simulink model "test_polbereichsvorgabe"  (R2016b)
settings: Solver=FixedStepAuto  StartTime=0.0  StopTime=20.0  FixedStep=1e-3  RelTol=1e-3
values from neighbouring files (symbols this model uses):
  A_11 = matA_g_u(1:numMessg,1:numMessg)    [calcRedBEO.m]
  A_12 = matA_g_u(1:numMessg,numMessg+1:end)    [calcRedBEO.m]
  A_21 = matA_g_u(numMessg+1:end,1:numMessg)    [calcRedBEO.m]
  A_22 = matA_g_u(numMessg+1:end,numMessg+1:end)    [calcRedBEO.m]
  A_D = -x(8)    [calc_regler_polbereichsvorgabe.m]
  B_1 = matB_g_u(1:numMessg)    [calcRedBEO.m]
  B_2 = matB_g_u(numMessg+1:end)    [calcRedBEO.m]
  B_D = [-x(5), -x(6), -x(7)]    [calc_regler_polbereichsvorgabe.m]
  C_D = x(4)    [calc_regler_polbereichsvorgabe.m]
  D_D = [x(1), x(2), x(3)]    [calc_regler_polbereichsvorgabe.m]
  matB = [0; (2*pi*sys.R*sys.K_K)/(sys.ue*sys.T_K); 0; (-2*pi*sys.R*sys.K_K)/(sys.ue*sys.T_K*sys.L)]    [calcSysMatrix.m]    (also in calcSysMatrixBEO.m = [0; (2*pi*sys.R*sys.K_K)/(sys.ue*sys.T_K)])
  matE = matB    [calcSysMatrix.m]    (also in calcSysMatrixBEO.m)
  matL = [l1 ... (first row only)    [calcRedBEO.m]
undefined symbols (not defined in the file or in its folder): system
libraries: simulink x2
settings Model: Creator=nicol  LastModifiedBy=nicol

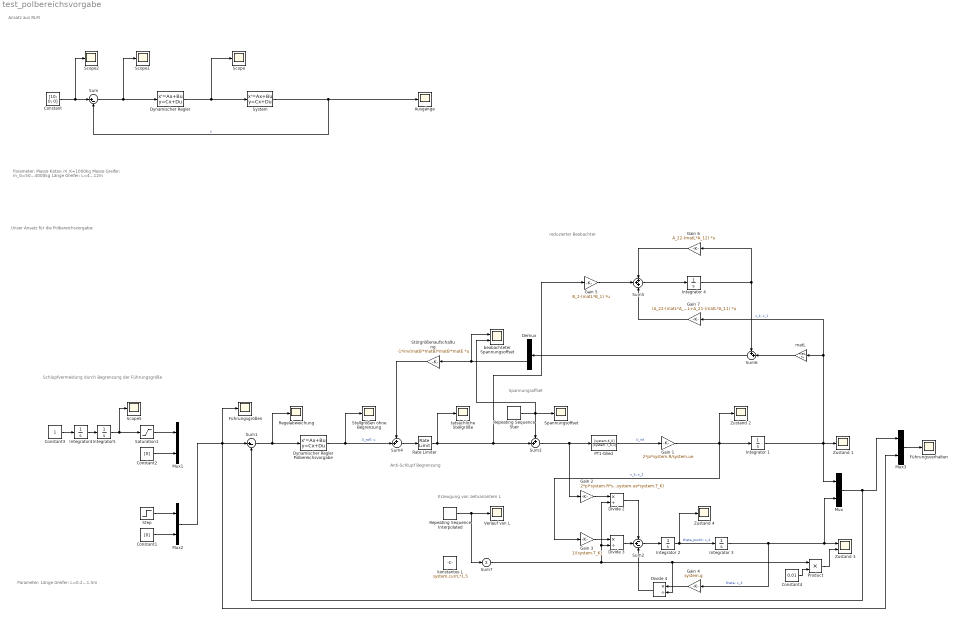
== system test_polbereichsvorgabe ==
  note: Erzeugung von zeitvariantem L
  note: reduzierter Beobachter
  note: Ansatz aus RLM
  note: Unser Ansatz für die Polbereichsvorgabe:
  note: Schlupfvermeidung durch Begrenzung
      | der Führungsgröße
  note: Parameter:
      | Masse Katze: m_K=1000kg
      | Masse Greifer: m_G=50...4000kg
      | Länge Greifer: L=4...12m
  note: Parameter:
      | Länge Greifer: L=0.2...1.5m
  note: Anti-Schlupf Begrenzung
  note: Spannungsoffset
  Ausgänge : Scope
  Constant : Constant  Value=[10; 0; 0]  VectorParams1D=off
  Constant1 : Constant  Value=[0]  VectorParams1D=off
  Constant2 : Constant  Value=[0]  VectorParams1D=off
  Constant3 : Constant
  Constant4 : Constant  Value=0.01
  Demux : Demux  Outputs=2
  Divide 2 : Product  Inputs=*/
  Divide 3 : Product  Inputs=*/
  Divide 4 : Product  Inputs=*/
  Dynamischer Regler : StateSpace  A=-0.6  B=[7.2 25.4 -306.2]  C=1000.7  D=[144.7 10294.8 -10032.5]  X0=0
  Dynamischer Regler Polbereichsvorgabe : StateSpace  A=A_D  B=-B_D  C=-C_D  D=D_D  X0=0
  Führungsgrößen : Scope
  Führungsverhalten : Scope
  Gain 1 : Gain  Gain=2*pi*system.R/system.ue
  Gain 2 : Gain  Gain=2*pi*system.R*system.K_K/(system.ue*system.T_K)
  Gain 3 : Gain  Gain=1/(system.T_K)
  Gain 4 : Gain  Gain=system.g
  Gain 5 : Gain  Gain=B_2-(matL*B_1)  Multiplication=Matrix(K*u)
  Gain 6 : Gain  Gain=A_22-(matL*A_12)  Multiplication=Matrix(K*u)
  Gain 7 : Gain  Gain=(A_22-(matL*A_12))*matL+A_21-(matL*A_11)  Multiplication=Matrix(K*u)
  Integrator {1..4} (4 alike) : Integrator
  Integrator4 : Integrator
  Integrator5 : Integrator
  Mux{,1..3} (4 alike) : Mux  Inputs=2
  PT1-Glied : TransferFcn  Numerator=[system.K_K]  Denominator=[system.T_K,1]
  Product : Product
  Rate Limiter : RateLimiter  RisingSlewLimit=4.32  FallingSlewLimit=-4.32  SampleTimeMode=inherited
  Regelabweichung : Scope
  Repeating Sequence Interpolated : simulink/Sources/Repeating Sequence Interpolated  OutValues=[1.5 1.0 0.7 0.5 0.4 0.3 0.2 0.5 1.5 1.0 0.2].'  TimeValues=[0 2 4 6 8 10 12 14 16 18 20].'  LookUpMeth=Interpolation-Use End Values  tsamp=0.01  OutMin=[]  OutMax=[]  OutDataTypeStr=double  OutputDataTypeScalingMode=double  OutDataType=fixdt(0,8)  OutScaling=2^-10
  Repeating Sequence Stair : simulink/Sources/Repeating Sequence Stair  OutValues=[0.2 0.1 0.05 0.2 0.1].'  tsamp=5  OutMin=[]  OutMax=[]  OutDataTypeStr=double  OutputDataTypeScalingMode=double  OutDataType=fixdt(0,8)  ConRadixGroup=Best Precision: Vector-wise  OutScaling=2^-12
  Saturation1 : Saturate  UpperLimit=2  LowerLimit=-2
  Scope{,1..2,5} (4 alike) : Scope
  Spannungsoffset : Scope
  Stellgrößen ohne Begrenzung : Scope
  Step : Step  After=2  SampleTime=0
  Störgrößenaufschaltung : Gain  Gain=-1*inv(matB'*matB)*matB'*matE  Multiplication=Matrix(K*u)
  Sum : Sum  Inputs=|+-
  Sum1 : Sum  Inputs=|+-
  Sum2 : Sum  Inputs=-+-
  Sum3 : Sum  Inputs=++|
  Sum4 : Sum  Inputs=++|
  Sum5 : Sum  Inputs=+++
  Sum6 : Sum  Inputs=++|
  Sum7 : Sum  Inputs=|+|
  System : StateSpace  A=[0 1 0 0; 0 0 39.24 0; 0 0 0 1; 0 0 -4.0875 0]  B=[0; 0.001; 0; -0.000083333]  C=[1 0 0 0; 0 1 0 0; 0 0 1 0]  D=[0; 0; 0]  X0=0
  Verlauf von L : Scope
  Zustand 1 : Scope
  Zustand 2 : Scope
  Zustand 3 : Scope  NumInputPorts=2
  Zustand 4 : Scope
  beobachteter Spannungsoffset : Scope  NumInputPorts=2
  konstantes L : Constant  Value=system.currL*1.5
  matL : Gain  Gain=matL  Multiplication=Matrix(K*u)
  tatsächliche Stellgröße : Scope
  wires:
  System/1 -> Sum/2, Ausgänge/1  "y"
  Constant/1 -> Scope2/1, Sum/1
  Dynamischer Regler/1 -> Scope/1, System/1
  Sum/1 -> Scope1/1, Dynamischer Regler/1
  Sum1/1 -> Dynamischer Regler Polbereichsvorgabe/1, Regelabweichung/1
  PT1-Glied/1 -> Gain 1/1  "U_ist"
  Gain 1/1 -> Zustand 2/1, Integrator 1/1, Gain 3/1  "v_k; x_2"
  Integrator 1/1 -> Gain 7/1, matL/1, Mux/1, Zustand 1/1  "x_k; x_1"
  Sum2/1 -> Integrator 2/1
  Integrator 2/1 -> Zustand 4/1, Integrator 3/1  "theta_punkt; x_4"
  Integrator 3/1 -> Gain 4/1, Mux/2, Zustand 3/1  "theta; x_3"
  Dynamischer Regler Polbereichsvorgabe/1 -> Sum4/2, Stellgrößen ohne Begrenzung/1  "U_soll; u"
  Mux/1 -> Mux3/1, Sum1/2
  Integrator4/1 -> Integrator5/1
  Integrator5/1 -> Saturation1/1, Scope5/1
  Constant3/1 -> Integrator4/1
  Saturation1/1 -> Mux1/1
  Constant2/1 -> Mux1/2
  Mux2/1 -> Mux3/2, Führungsgrößen/1, Sum1/1
  Constant1/1 -> Mux2/2
  Step/1 -> Mux2/1
  Mux3/1 -> Führungsverhalten/1
  Sum3/1 -> Gain 2/1, PT1-Glied/1
  Repeating Sequence Stair/1 -> beobachteter Spannungsoffset/2, Spannungsoffset/1, Sum3/1
  Sum4/1 -> Rate Limiter/1
  Gain 5/1 -> Sum5/2
  Sum5/1 -> Integrator 4/1
  Gain 6/1 -> Sum5/1
  Gain 7/1 -> Sum5/3
  matL/1 -> Sum6/2
  Integrator 4/1 -> Sum6/1, Gain 6/1
  Sum6/1 -> Demux/1
  Rate Limiter/1 -> Gain 5/1, Sum3/2, tatsächliche Stellgröße/1
  Störgrößenaufschaltung/1 -> Sum4/1
  Repeating Sequence Interpolated/1 -> Sum7/1, Verlauf von L/1
  Gain 2/1 -> Divide 2/1
  Divide 2/1 -> Sum2/1
  Gain 3/1 -> Divide 3/1
  Divide 3/1 -> Sum2/2
  Gain 4/1 -> Divide 4/1
  Divide 4/1 -> Sum2/3
  Sum7/1 -> Divide 3/2, Divide 2/2, Product/1, Divide 4/2
  Demux/2 -> beobachteter Spannungsoffset/1, Störgrößenaufschaltung/1
  Product/1 -> Zustand 3/2
  Constant4/1 -> Product/2
